simulink model "Test_N1"  (R2020b)
settings: Solver=ode3  StartTime=0.0  StopTime=inf  FixedStep=0.05  RelTol=1e-3
libraries: Utilities x3, Sensors x2, XBotBlockToolbox x2

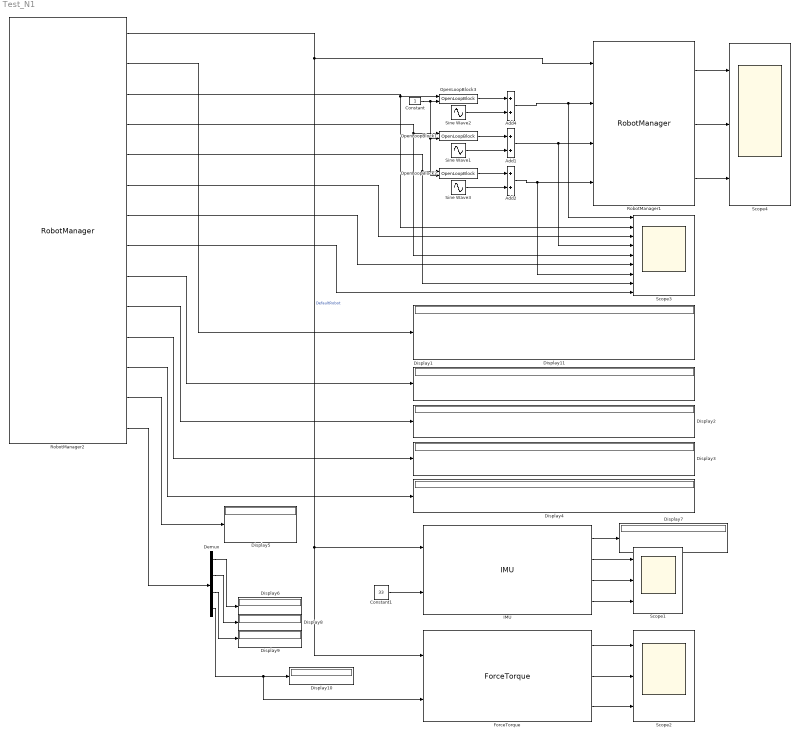
== system Test_N1 ==
  Add1 : Sum
  Add2 : Sum
  Add4 : Sum
  Constant : Constant
  Constant1 : Constant  Value=33
  Demux : Demux
  Display{1..11} (11 alike) : Display
  ForceTorque : Sensors/ForceTorque  ManagerName=DefaultRobot  ManagerType=Robot  ForceTorqueList={ 'f', 't', 'w' }
  IMU : Sensors/IMU  ManagerName=DefaultRobot  ManagerType=Robot  IMUList={ 'orient', 'quat', 'a', 'omega' }
  OpenLoopBlock1 : Utilities/OpenLoopBlock  SystemSampleTime=-1  VariantActivationTime=update diagram  Latency=0  AutoFrameSizeCalculation=off
  OpenLoopBlock2 : Utilities/OpenLoopBlock  SystemSampleTime=-1  VariantActivationTime=update diagram  Latency=0  AutoFrameSizeCalculation=off
  OpenLoopBlock3 : Utilities/OpenLoopBlock  SystemSampleTime=-1  VariantActivationTime=update diagram  Latency=0  AutoFrameSizeCalculation=off
  RobotManager1 : XBotBlockToolbox/RobotManager  RobotName=DefaultRobot  ModelName=DefaultRobot  UseExtRobot=On  SyncWithModel=Off  ReadingsList={}  MechanicalLimitsList={}  MechanicalLimitsCheck=On  MechanicalLimitsEnforce=On  SensorList={}  ReferencesList={ 'qJ_ref', 'qJdot_ref', 'tau_ref' }  OldRobotName=DefaultRobot
  RobotManager2 : XBotBlockToolbox/RobotManager  RobotName=DefaultRobot  ModelName=DefaultModel  UseExtRobot=Off  SyncWithModel=Off  ReadingsList={ 'q_ID', 'qJ', 'qJdot', 'tau', 'qJ_ref', 'qJdot_ref', 'tau_ref' }  MechanicalLimitsList={ 'q_min', 'q_max', 'qdot_max', 'tau_max' }  MechanicalLimitsCheck=Off  MechanicalLimitsEnforce=Off  SensorList={ 'IMU', 'FT' }  ReferencesList={}  OldRobotName=DefaultRobot
  Scope1 : Scope  NumInputPorts=3
  Scope2 : Scope  NumInputPorts=3
  Scope3 : Scope  NumInputPorts=9
  Scope4 : Scope  NumInputPorts=3
  Sine Wave1 : Sin  Amplitude=10  SampleTime=0
  Sine Wave2 : Sin  Amplitude=0.2  SampleTime=0
  Sine Wave3 : Sin  Amplitude=300  SampleTime=0
  wires:
  RobotManager2/1 -> IMU/1, ForceTorque/1, RobotManager1/1  "DefaultRobot"
  OpenLoopBlock3/1 -> Add4/1
  RobotManager2/9 -> Display1/1
  RobotManager2/10 -> Display2/1
  RobotManager2/11 -> Display3/1
  RobotManager2/12 -> Display4/1
  Sine Wave2/1 -> Add4/2
  RobotManager2/3 -> Scope3/2, OpenLoopBlock3/1
  OpenLoopBlock1/1 -> Add1/1
  RobotManager2/4 -> Scope3/5, OpenLoopBlock1/1
  Sine Wave1/1 -> Add1/2
  OpenLoopBlock2/1 -> Add2/1
  RobotManager2/5 -> Scope3/8, OpenLoopBlock2/1
  Sine Wave3/1 -> Add2/2
  Add4/1 -> Scope3/1, RobotManager1/2
  Add1/1 -> Scope3/4, RobotManager1/3
  Add2/1 -> Scope3/7, RobotManager1/4
  RobotManager2/6 -> Scope3/3
  RobotManager2/7 -> Scope3/6
  RobotManager2/8 -> Scope3/9
  Constant/1 -> OpenLoopBlock1/2, OpenLoopBlock2/2, OpenLoopBlock3/2
  IMU/1 -> Display7/1
  IMU/2 -> Scope1/1
  IMU/3 -> Scope1/2
  IMU/4 -> Scope1/3
  ForceTorque/2 -> Scope2/2
  ForceTorque/1 -> Scope2/1
  ForceTorque/3 -> Scope2/3
  RobotManager2/13 -> Display5/1
  Demux/1 -> Display6/1
  Demux/2 -> Display8/1
  Demux/3 -> Display9/1
  Demux/4 -> ForceTorque/2, Display10/1
  RobotManager2/14 -> Demux/1
  Constant1/1 -> IMU/2
  RobotManager1/1 -> Scope4/1
  RobotManager1/2 -> Scope4/2
  RobotManager1/3 -> Scope4/3
  RobotManager2/2 -> Display11/1
